simulink model "pendulum_simulation"  (R2023b)
settings: Solver=VariableStepAuto  StartTime=0.0  StopTime=100  RelTol=1e-3
settings Model: Creator=davidbombara  LastModifiedBy=davidbombara

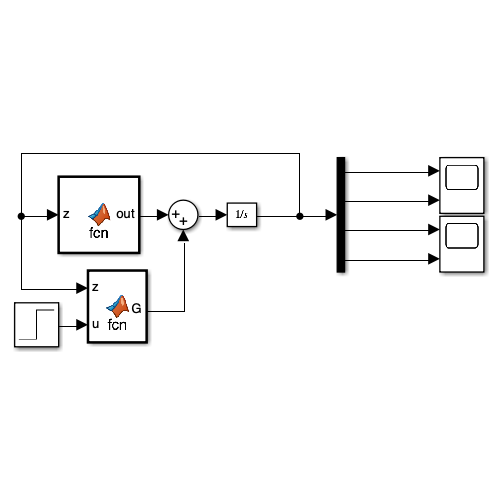
[thumbnail: Simulink's stored preview of the top-level diagram]
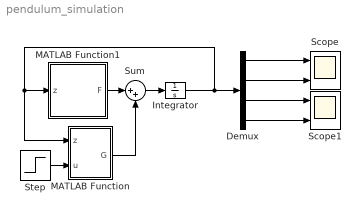
== system pendulum_simulation ==
  Demux : Demux
  Integrator : Integrator  InitialCondition=[pi;0;10;10]
  MATLAB Function : MATLAB Function  TreatAsAtomicUnit=on
  MATLAB Function1 : MATLAB Function  TreatAsAtomicUnit=on
  Scope : Scope  NumInputPorts=2
  Scope1 : Scope  NumInputPorts=2
  Step : Step  SampleTime=0
  Sum : Sum  Inputs=|++
  wires:
  Sum/1 -> Integrator/1
  MATLAB Function/1(G) -> Sum/2
  Integrator/1 -> Demux/1, MATLAB Function/1(z), MATLAB Function1/1(z)
  Step/1 -> MATLAB Function/2(u)
  Demux/1 -> Scope/1
  Demux/2 -> Scope/2
  Demux/4 -> Scope1/2
  Demux/3 -> Scope1/1
  MATLAB Function1/1(F) -> Sum/1

== matlab function pendulum_simulation/MATLAB Function ==
  data: z input; u input; G output
function G = fcn(z,u)
    b = 0.1;m = 1;g = 9.8;l = 1;
    B = [0; (u - m*g*l*sin(z(1)))/(m*l^2)];
    G = [B;0;0];

== matlab function pendulum_simulation/MATLAB Function1 ==
  data: z input; F output
function F = fcn(z)
    b = 0.1;m = 1;g = 9.8;l = 1;
    A = [0,1; 0, -b/(m*l^2)];
    k1 = 0.2006;k2 = 0.4985;
    C = [1,0];
    K = [k1;k2];
    F = [A,zeros(2,2);zeros(2,2),(A - K*C)]*z;
